simulink model "Controllers"  (R2022b)
settings: Solver=FixedStepAuto  StartTime=0.0  StopTime=60  FixedStep=.01  RelTol=1e-3
values from neighbouring files (symbols this model uses):
  g = [0, 0, 1]    [myMeasurementFcn.m]    (also in test_DELETE.m = [0,0,0,1])
undefined symbols (not defined in the file or in its folder): CdProp, Ct, larm, mass
libraries: slpidlib x6, sharedtransform x2
settings Model: Creator=aaron  LastModifiedBy=aaron
settings DataIOCC: SaveOutput=off  SaveTime=off
settings DebuggingCC: ModelReferenceExtraNoncontSigs=none

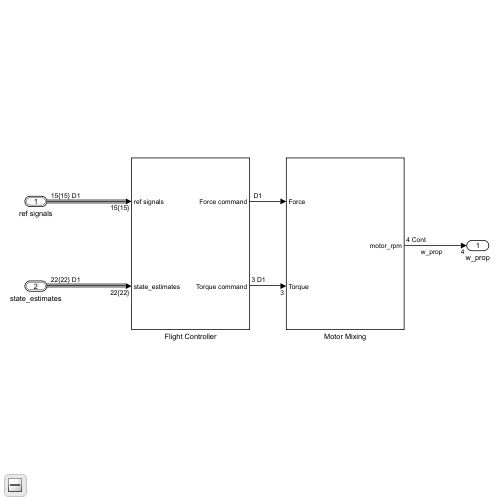
[thumbnail: Simulink's stored preview of the top-level diagram]
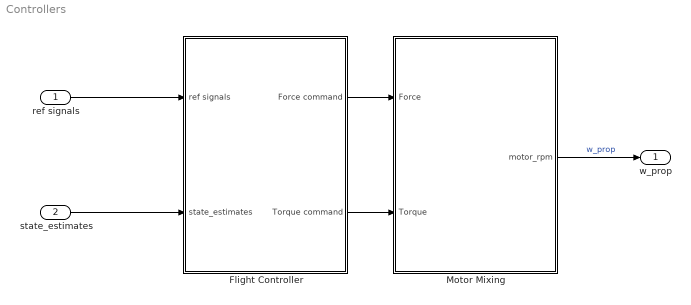
== system Controllers ==
  ref signals : Inport  OutDataTypeStr=Bus: reference_signals  SampleTime=[.01,0]  LockScale=on
  state_estimates : Inport  Port=2  OutDataTypeStr=Bus: state_estimates  SampleTime=[.01,0]  LockScale=on
  Flight Controller : Subsystem
  Motor Mixing : Subsystem
  w_prop : Outport  OutDataTypeStr=single  PortDimensions=4  SampleTime=0
  wires:
  state_estimates/1 -> Flight Controller/2(state_estimates)
  Motor Mixing/1(motor_rpm) -> w_prop/1  "w_prop"
  ref signals/1 -> Flight Controller/1(ref signals)
  Flight Controller/2(Torque command) -> Motor Mixing/2(Torque)
  Flight Controller/1(Force command) -> Motor Mixing/1(Force)

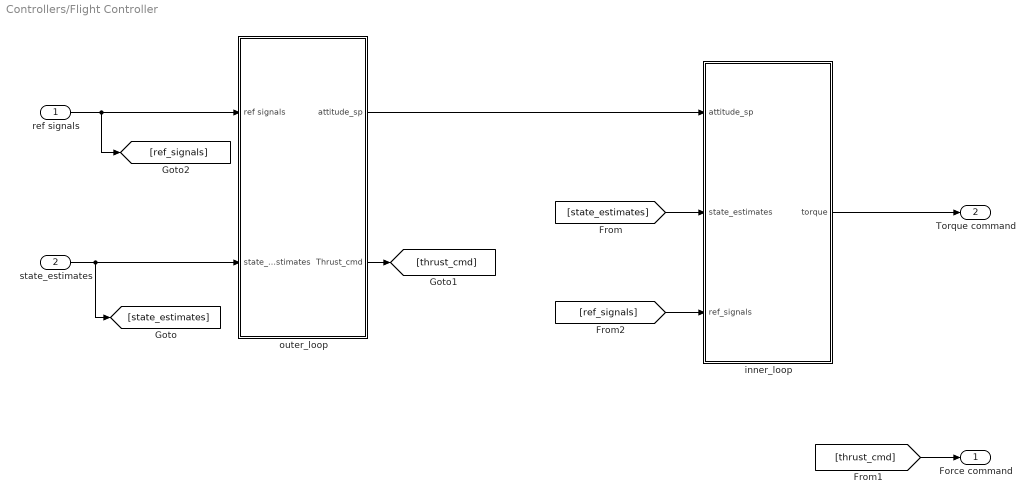
== system Controllers/Flight Controller ==
  ref signals : Inport  OutDataTypeStr=Bus: reference_signals  SampleTime=[.01,0]  LockScale=on
  state_estimates : Inport  Port=2  OutDataTypeStr=Bus: state_estimates  SampleTime=[.01,0]  LockScale=on
  inner_loop : Subsystem
  outer_loop : Subsystem
  Force command : Outport
  Torque command : Outport  Port=2
  wires:
  state_estimates/1 -> outer_loop/2(state_estimates), [state_estimates]
  ref signals/1 -> [ref_signals], outer_loop/1(ref signals)
  outer_loop/1(attitude_sp) -> inner_loop/1(attitude_sp)
  [state_estimates] -> inner_loop/2(state_estimates)
  inner_loop/1(torque) -> Torque command/1
  outer_loop/2(Thrust_cmd) -> [thrust_cmd]
  [thrust_cmd] -> Force command/1
  [ref_signals] -> inner_loop/3(ref_signals)

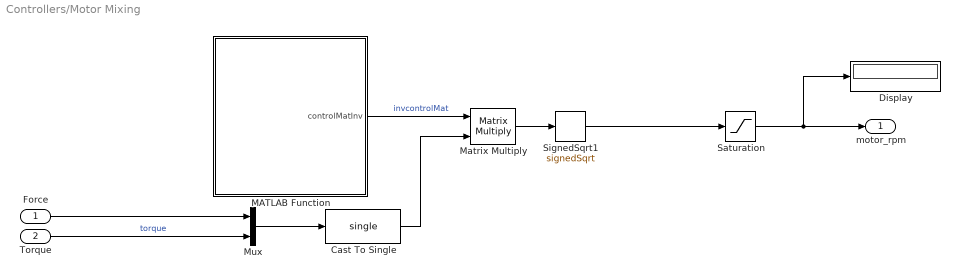
== system Controllers/Motor Mixing ==
  Force : Inport
  Torque : Inport  Port=2
  Cast To Single : DataTypeConversion  OutDataTypeStr=single  SaturateOnIntegerOverflow=off  RndMeth=Floor
  Display : Display
  MATLAB Function : MATLAB Function  TreatAsAtomicUnit=on
  Matrix Multiply : Product  Multiplication=Matrix(*)
  Mux : Mux  Inputs=2
  Saturation : Saturate  UpperLimit=2000  LowerLimit=0
  SignedSqrt1 : Sqrt  Operator=signedSqrt  IntermediateResultsDataTypeStr=single
  motor_rpm : Outport
  wires:
  Torque/1 -> Mux/2  "torque"
  Force/1 -> Mux/1
  Saturation/1 -> Display/1, motor_rpm/1
  SignedSqrt1/1 -> Saturation/1
  Matrix Multiply/1 -> SignedSqrt1/1
  MATLAB Function/1(controlMatInv) -> Matrix Multiply/1  "invcontrolMat"
  Cast To Single/1 -> Matrix Multiply/2
  Mux/1 -> Cast To Single/1

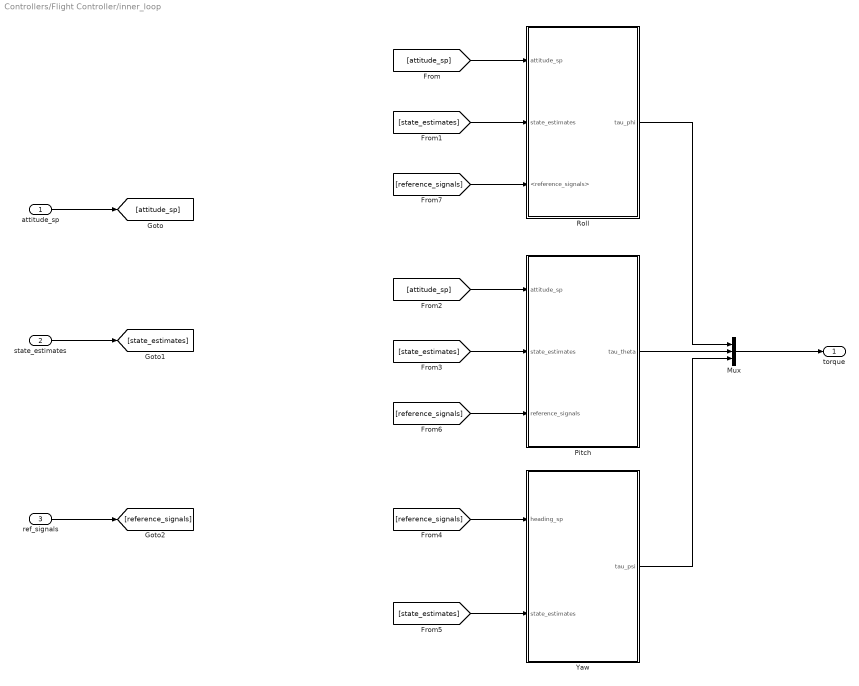
== system Controllers/Flight Controller/inner_loop ==
  attitude_sp : Inport
  state_estimates : Inport  Port=2  OutDataTypeStr=Bus: state_estimates  SampleTime=[.01,0]
  ref_signals : Inport  Port=3  OutDataTypeStr=Bus: reference_signals  SampleTime=[.01,0]
  Mux : Mux  Inputs=3
  Pitch : Subsystem
  Roll : Subsystem
  Yaw : Subsystem
  torque : Outport
  wires:
  [reference_signals] -> Roll/3(<reference_signals>)
  [reference_signals] -> Pitch/3(reference_signals)
  [reference_signals] -> Yaw/1(heading_sp)
  ref_signals/1 -> [reference_signals]
  attitude_sp/1 -> [attitude_sp]
  state_estimates/1 -> [state_estimates]
  [attitude_sp] -> Roll/1(attitude_sp)
  [state_estimates] -> Roll/2(state_estimates)
  [attitude_sp] -> Pitch/1(attitude_sp)
  [state_estimates] -> Pitch/2(state_estimates)
  [state_estimates] -> Yaw/2(state_estimates)
  Roll/1(tau_phi) -> Mux/1
  Mux/1 -> torque/1
  Pitch/1(tau_theta) -> Mux/2
  Yaw/1(tau_psi) -> Mux/3

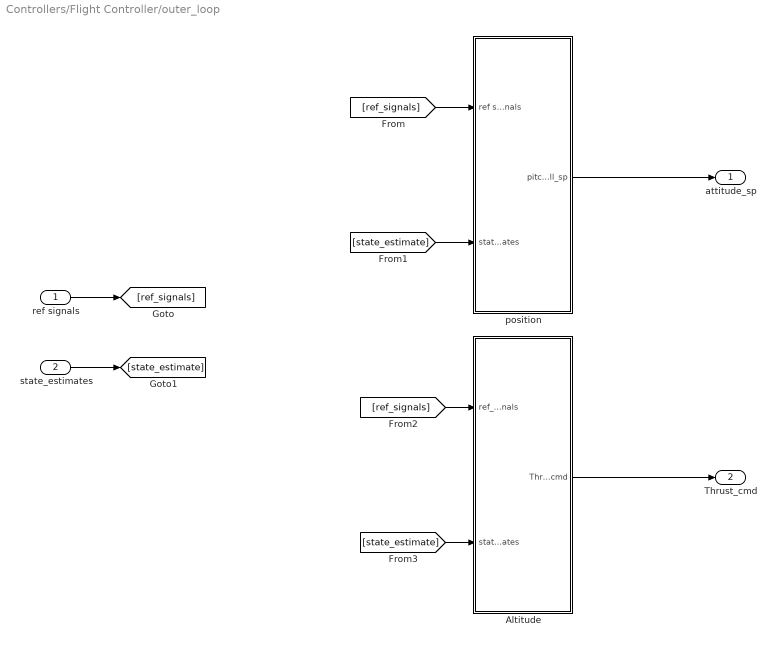
== system Controllers/Flight Controller/outer_loop ==
  ref signals : Inport  OutDataTypeStr=Bus: reference_signals  LockScale=on
  state_estimates : Inport  Port=2  OutDataTypeStr=Bus: state_estimates  LockScale=on
  Altitude : Subsystem
  position : Subsystem
  attitude_sp : Outport
  Thrust_cmd : Outport  Port=2
  wires:
  position/1(pitch_roll_sp) -> attitude_sp/1
  Altitude/1(Thrust_cmd) -> Thrust_cmd/1
  ref signals/1 -> [ref_signals]
  state_estimates/1 -> [state_estimate]
  [ref_signals] -> position/1(ref signals)
  [state_estimate] -> position/2(state_estimates)
  [ref_signals] -> Altitude/1(ref_signals)
  [state_estimate] -> Altitude/2(state_estimates)

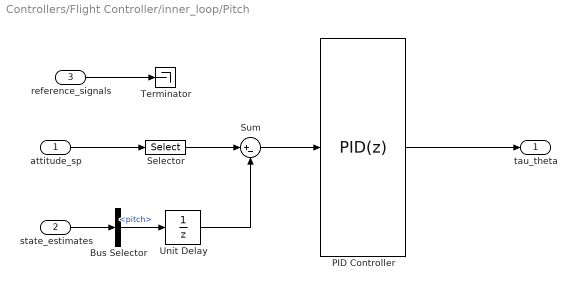
== system Controllers/Flight Controller/inner_loop/Pitch ==
  attitude_sp : Inport
  state_estimates : Inport  Port=2  OutDataTypeStr=Bus: state_estimates  SampleTime=[.01,0]
  reference_signals : Inport  Port=3  OutDataTypeStr=Bus: reference_signals  SampleTime=[.01,0]
  Bus Selector : BusSelector  OutputSignals=euler.pitch
  PID Controller : slpidlib/PID Controller  Controller=PID  Form=Parallel  TimeDomain=Discrete-time  UseExternalTs=off  SampleTime=-1  IntegratorMethod=Forward Euler  FilterMethod=Forward Euler  ControllerParametersSource=internal  P=0.000755  I=1.95e-05  UseKiTs=off  D=0.00509  N=1.0382  UseFilter=on  TunerSelectOption=Transfer Function Based (PID Tuner App)  InitialConditionSource=internal  InitialConditionForIntegrator=0  InitialConditionForFilter=0  DifferentiatorICPrevScaledInput=0  ExternalReset=none  TrackingMode=off  Kt=1  LimitOutput=off  SatLimitsSource=internal  UpperSaturationLimit=inf  LowerSaturationLimit=-inf  LinearizeAsGain=on  AntiWindupMode=clamping  Kb=1  LimitIntegrator=off  UpperIntegratorSaturationLimit=inf  LowerIntegratorSaturationLimit=-inf  POutMin=[]  POutMax=[]  IOutMin=[]  IOutMax=[]  DOutMin=[]  DOutMax=[]  NOutMin=[]  NOutMax=[]  SumOutMin=[]  SumOutMax=[]  SaturationOutMin=[]  SaturationOutMax=[]  PParamMin=[]  PParamMax=[]  IParamMin=[]  IParamMax=[]  DParamMin=[]  DParamMax=[]  NParamMin=[]  NParamMax=[]  KbParamMin=[]  KbParamMax=[]  KtParamMin=[]  KtParamMax=[]  KbOutMin=[]  KbOutMax=[]  KtOutMin=[]  KtOutMax=[]  IntegratorOutMin=[]  IntegratorOutMax=[]  FilterOutMin=[]  FilterOutMax=[]  SumI1OutMin=[]  SumI1OutMax=[]  SumI2OutMin=[]  SumI2OutMax=[]  SumI3OutMin=[]  SumI3OutMax=[]  SumI4OutMin=[]  SumI4OutMax=[]  SumDOutMin=[]  SumDOutMax=[]  DifferentiatorOutMin=[]  DifferentiatorOutMax=[]  FilterDiffOutCoefMin=[]  FilterDiffOutCoefMax=[]  ReciprocalOutMin=[]  ReciprocalOutMax=[]  SumDenOutMin=[]  SumDenOutMax=[]  SumNumOutMin=[]  SumNumOutMax=[]  DivideOutMin=[]  DivideOutMax=[]  UdiffTsProdOutMin=[]  UdiffTsProdOutMax=[]  NTsProdOutMin=[]  NTsProdOutMax=[]  UintegralTsProdOutMin=[]  UintegralTsProdOutMax=[]  UngainTsProdOutMin=[]  UngainTsProdOutMax=[]  ClampingZeroOutDataTypeStr=Inherit: Inherit via back propagation  ClampingZeroOutMin=[]  ClampingZeroOutMax=[]  FilterDenConstantOutDataTypeStr=Inherit: Inherit via back propagation  FilterDenConstantOutMin=[]  FilterDenConstantOutMax=[]  PCopyOutDataTypeStr=Inherit: Inherit via back propagation  PCopyOutMin=[]  PCopyOutMax=[]  NCopyOutDataTypeStr=Inherit: Inherit via back propagation  NCopyOutMin=[]  NCopyOutMax=[]  IntegratorContinuousStateAttributes=''  IntegratorStateMustResolveToSignalObject=off  IntegratorRTWStateStorageClass=Auto  FilterContinuousStateAttributes=''  FilterStateMustResolveToSignalObject=off  FilterRTWStateStorageClass=Auto  ParallelPVariant=InternalParameters  IdealPVariant=Disabled  IVariant=InternalParameters  DVariant=InternalParameters  IntegratorVariant=Discrete  SatVariant=Disabled  AWVariant=Passthrough  PCopyVariant=Disabled  TRVariant=Disabled  FdbkBlocksVariant=Forward  IdealPFdbkVariant=Disabled  SatFdbkVariant=Disabled  DerivativeFilterVariant=ForwardEulerFilter  NVariant=InternalParameters  NCopyVariant=Disabled  FilterICVariant=InternalICsFilter  IntegratorICVariant=InternalICs  ExternalResetVariant=Disabled  TRSumVariant=Passthrough  SumFdbkVariant=Disabled  SumVariant=Sum_PID  TsampFilterVariant=InternalTs  TsampNgainVariant=Passthrough  TsampIntegralVariant=Passthrough  ExternalSaturationOutDataTypeStr=Inherit: Same as second input
  Selector : Selector  InputPortWidth=2  IndexOptions=Index vector (dialog)  Indices=[2]  OutputSizes=1
  Sum : Sum  Inputs=|+-
  Terminator : Terminator
  Unit Delay : UnitDelay  InitialCondition=single(0)  SampleTime=-1  HasFrameUpgradeWarning=on
  tau_theta : Outport
  wires:
  attitude_sp/1 -> Selector/1
  Sum/1 -> PID Controller/1
  PID Controller/1 -> tau_theta/1
  Bus Selector/1 -> Unit Delay/1  "<pitch>"
  state_estimates/1 -> Bus Selector/1
  reference_signals/1 -> Terminator/1
  Selector/1 -> Sum/1
  Unit Delay/1 -> Sum/2

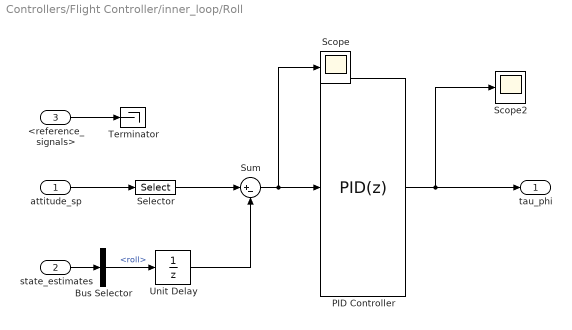
== system Controllers/Flight Controller/inner_loop/Roll ==
  attitude_sp : Inport
  state_estimates : Inport  Port=2  OutDataTypeStr=Bus: state_estimates
  <reference_signals> : Inport  Port=3  OutDataTypeStr=Bus: reference_signals
  Bus Selector : BusSelector  OutputSignals=euler.roll
  PID Controller : slpidlib/PID Controller  Controller=PID  Form=Parallel  TimeDomain=Discrete-time  UseExternalTs=off  SampleTime=-1  IntegratorMethod=Forward Euler  FilterMethod=Forward Euler  ControllerParametersSource=internal  P=0.00222776202264695  I=2.18485015437245e-05  UseKiTs=off  D=0.0134340999324703  N=1.24748629813611  UseFilter=on  TunerSelectOption=Transfer Function Based (PID Tuner App)  InitialConditionSource=internal  InitialConditionForIntegrator=0  InitialConditionForFilter=0  DifferentiatorICPrevScaledInput=0  ExternalReset=none  TrackingMode=off  Kt=1  LimitOutput=off  SatLimitsSource=internal  UpperSaturationLimit=inf  LowerSaturationLimit=-inf  LinearizeAsGain=on  AntiWindupMode=clamping  Kb=1  LimitIntegrator=off  UpperIntegratorSaturationLimit=inf  LowerIntegratorSaturationLimit=-inf  POutMin=[]  POutMax=[]  IOutMin=[]  IOutMax=[]  DOutMin=[]  DOutMax=[]  NOutMin=[]  NOutMax=[]  SumOutMin=[]  SumOutMax=[]  SaturationOutMin=[]  SaturationOutMax=[]  PParamMin=[]  PParamMax=[]  IParamMin=[]  IParamMax=[]  DParamMin=[]  DParamMax=[]  NParamMin=[]  NParamMax=[]  KbParamMin=[]  KbParamMax=[]  KtParamMin=[]  KtParamMax=[]  KbOutMin=[]  KbOutMax=[]  KtOutMin=[]  KtOutMax=[]  IntegratorOutMin=[]  IntegratorOutMax=[]  FilterOutMin=[]  FilterOutMax=[]  SumI1OutMin=[]  SumI1OutMax=[]  SumI2OutMin=[]  SumI2OutMax=[]  SumI3OutMin=[]  SumI3OutMax=[]  SumI4OutMin=[]  SumI4OutMax=[]  SumDOutMin=[]  SumDOutMax=[]  DifferentiatorOutMin=[]  DifferentiatorOutMax=[]  FilterDiffOutCoefMin=[]  FilterDiffOutCoefMax=[]  ReciprocalOutMin=[]  ReciprocalOutMax=[]  SumDenOutMin=[]  SumDenOutMax=[]  SumNumOutMin=[]  SumNumOutMax=[]  DivideOutMin=[]  DivideOutMax=[]  UdiffTsProdOutMin=[]  UdiffTsProdOutMax=[]  NTsProdOutMin=[]  NTsProdOutMax=[]  UintegralTsProdOutMin=[]  UintegralTsProdOutMax=[]  UngainTsProdOutMin=[]  UngainTsProdOutMax=[]  ClampingZeroOutDataTypeStr=Inherit: Inherit via back propagation  ClampingZeroOutMin=[]  ClampingZeroOutMax=[]  FilterDenConstantOutDataTypeStr=Inherit: Inherit via back propagation  FilterDenConstantOutMin=[]  FilterDenConstantOutMax=[]  PCopyOutDataTypeStr=Inherit: Inherit via back propagation  PCopyOutMin=[]  PCopyOutMax=[]  NCopyOutDataTypeStr=Inherit: Inherit via back propagation  NCopyOutMin=[]  NCopyOutMax=[]  IntegratorContinuousStateAttributes=''  IntegratorStateMustResolveToSignalObject=off  IntegratorRTWStateStorageClass=Auto  FilterContinuousStateAttributes=''  FilterStateMustResolveToSignalObject=off  FilterRTWStateStorageClass=Auto  ParallelPVariant=InternalParameters  IdealPVariant=Disabled  IVariant=InternalParameters  DVariant=InternalParameters  IntegratorVariant=Discrete  SatVariant=Disabled  AWVariant=Passthrough  PCopyVariant=Disabled  TRVariant=Disabled  FdbkBlocksVariant=Forward  IdealPFdbkVariant=Disabled  SatFdbkVariant=Disabled  DerivativeFilterVariant=ForwardEulerFilter  NVariant=InternalParameters  NCopyVariant=Disabled  FilterICVariant=InternalICsFilter  IntegratorICVariant=InternalICs  ExternalResetVariant=Disabled  TRSumVariant=Passthrough  SumFdbkVariant=Disabled  SumVariant=Sum_PID  TsampFilterVariant=InternalTs  TsampNgainVariant=Passthrough  TsampIntegralVariant=Passthrough  ExternalSaturationOutDataTypeStr=Inherit: Same as second input
  Scope : Scope
  Scope2 : Scope
  Selector : Selector  InputPortWidth=2  IndexOptions=Index vector (dialog)  Indices=[1]  OutputSizes=1
  Sum : Sum  Inputs=|+-
  Terminator : Terminator
  Unit Delay : UnitDelay  InitialCondition=single(0)  SampleTime=-1  HasFrameUpgradeWarning=on
  tau_phi : Outport
  wires:
  attitude_sp/1 -> Selector/1
  Sum/1 -> PID Controller/1, Scope/1
  PID Controller/1 -> Scope2/1, tau_phi/1
  state_estimates/1 -> Bus Selector/1
  Bus Selector/1 -> Unit Delay/1  "<roll>"
  <reference_signals>/1 -> Terminator/1
  Selector/1 -> Sum/1
  Unit Delay/1 -> Sum/2

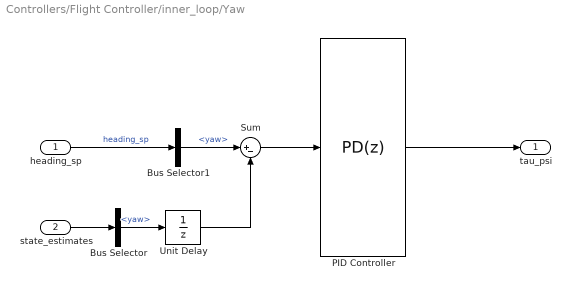
== system Controllers/Flight Controller/inner_loop/Yaw ==
  heading_sp : Inport  OutDataTypeStr=Bus: reference_signals
  state_estimates : Inport  Port=2  OutDataTypeStr=Bus: state_estimates
  Bus Selector : BusSelector  OutputSignals=euler.yaw
  Bus Selector1 : BusSelector  OutputSignals=euler.yaw
  PID Controller : slpidlib/PID Controller  Controller=PD  Form=Parallel  TimeDomain=Discrete-time  UseExternalTs=off  SampleTime=-1  IntegratorMethod=Forward Euler  FilterMethod=Forward Euler  ControllerParametersSource=internal  P=0.00308709400862221  I=0  UseKiTs=off  D=0.020762699011989  N=9.31948574377754  UseFilter=on  TunerSelectOption=Transfer Function Based (PID Tuner App)  InitialConditionSource=internal  InitialConditionForIntegrator=0  InitialConditionForFilter=0  DifferentiatorICPrevScaledInput=0  ExternalReset=none  TrackingMode=off  Kt=1  LimitOutput=off  SatLimitsSource=internal  UpperSaturationLimit=inf  LowerSaturationLimit=-inf  LinearizeAsGain=on  AntiWindupMode=clamping  Kb=1  LimitIntegrator=off  UpperIntegratorSaturationLimit=inf  LowerIntegratorSaturationLimit=-inf  POutMin=[]  POutMax=[]  IOutMin=[]  IOutMax=[]  DOutMin=[]  DOutMax=[]  NOutMin=[]  NOutMax=[]  SumOutMin=[]  SumOutMax=[]  SaturationOutMin=[]  SaturationOutMax=[]  PParamMin=[]  PParamMax=[]  IParamMin=[]  IParamMax=[]  DParamMin=[]  DParamMax=[]  NParamMin=[]  NParamMax=[]  KbParamMin=[]  KbParamMax=[]  KtParamMin=[]  KtParamMax=[]  KbOutMin=[]  KbOutMax=[]  KtOutMin=[]  KtOutMax=[]  IntegratorOutMin=[]  IntegratorOutMax=[]  FilterOutMin=[]  FilterOutMax=[]  SumI1OutMin=[]  SumI1OutMax=[]  SumI2OutMin=[]  SumI2OutMax=[]  SumI3OutMin=[]  SumI3OutMax=[]  SumI4OutMin=[]  SumI4OutMax=[]  SumDOutMin=[]  SumDOutMax=[]  DifferentiatorOutMin=[]  DifferentiatorOutMax=[]  FilterDiffOutCoefMin=[]  FilterDiffOutCoefMax=[]  ReciprocalOutMin=[]  ReciprocalOutMax=[]  SumDenOutMin=[]  SumDenOutMax=[]  SumNumOutMin=[]  SumNumOutMax=[]  DivideOutMin=[]  DivideOutMax=[]  UdiffTsProdOutMin=[]  UdiffTsProdOutMax=[]  NTsProdOutMin=[]  NTsProdOutMax=[]  UintegralTsProdOutMin=[]  UintegralTsProdOutMax=[]  UngainTsProdOutMin=[]  UngainTsProdOutMax=[]  ClampingZeroOutDataTypeStr=Inherit: Inherit via back propagation  ClampingZeroOutMin=[]  ClampingZeroOutMax=[]  FilterDenConstantOutDataTypeStr=Inherit: Inherit via back propagation  FilterDenConstantOutMin=[]  FilterDenConstantOutMax=[]  PCopyOutDataTypeStr=Inherit: Inherit via back propagation  PCopyOutMin=[]  PCopyOutMax=[]  NCopyOutDataTypeStr=Inherit: Inherit via back propagation  NCopyOutMin=[]  NCopyOutMax=[]  IntegratorContinuousStateAttributes=''  IntegratorStateMustResolveToSignalObject=off  IntegratorRTWStateStorageClass=Auto  FilterContinuousStateAttributes=''  FilterStateMustResolveToSignalObject=off  FilterRTWStateStorageClass=Auto  ParallelPVariant=InternalParameters  IdealPVariant=Disabled  IVariant=Disabled  DVariant=InternalParameters  IntegratorVariant=Disabled  SatVariant=Disabled  AWVariant=Disabled  PCopyVariant=Disabled  TRVariant=Disabled  FdbkBlocksVariant=Forward  IdealPFdbkVariant=Disabled  SatFdbkVariant=Disabled  DerivativeFilterVariant=ForwardEulerFilter  NVariant=InternalParameters  NCopyVariant=Disabled  FilterICVariant=InternalICsFilter  IntegratorICVariant=Disabled  ExternalResetVariant=Disabled  TRSumVariant=Passthrough  SumFdbkVariant=Disabled  SumVariant=Sum_PD  TsampFilterVariant=InternalTs  TsampNgainVariant=Passthrough  TsampIntegralVariant=Disabled_SignalSpec  ExternalSaturationOutDataTypeStr=Inherit: Same as second input
  Sum : Sum  Inputs=|+-
  Unit Delay : UnitDelay  InitialCondition=single(0)  SampleTime=-1  HasFrameUpgradeWarning=on
  tau_psi : Outport
  wires:
  heading_sp/1 -> Bus Selector1/1  "heading_sp"
  Bus Selector1/1 -> Sum/1  "<yaw>"
  PID Controller/1 -> tau_psi/1
  Bus Selector/1 -> Unit Delay/1  "<yaw>"
  state_estimates/1 -> Bus Selector/1
  Sum/1 -> PID Controller/1
  Unit Delay/1 -> Sum/2

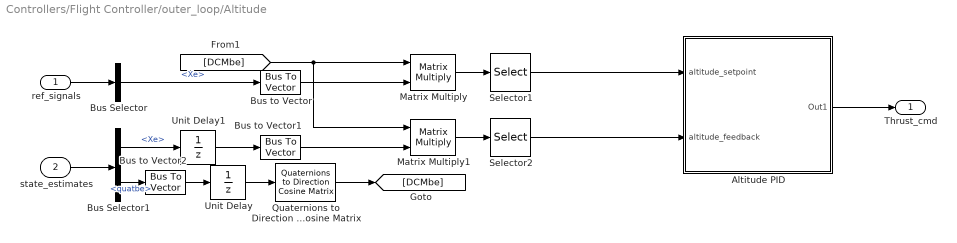
== system Controllers/Flight Controller/outer_loop/Altitude ==
  ref_signals : Inport  OutDataTypeStr=Bus: reference_signals  SampleTime=[.01,0]
  state_estimates : Inport  Port=2  OutDataTypeStr=Bus: state_estimates  SampleTime=[.01,0]
  Altitude PID : Subsystem
  Bus Selector : BusSelector  OutputSignals=Xe
  Bus Selector1 : BusSelector  OutputSignals=Xe,quatbe
  Bus to Vector : BusToVector
  Bus to Vector1 : BusToVector
  Bus to Vector2 : BusToVector
  Matrix Multiply : Product  Multiplication=Matrix(*)
  Matrix Multiply1 : Product  Multiplication=Matrix(*)
  Quaternions to Direction Cosine Matrix : sharedtransform/Quaternions to  Direction Cosine Matrix  aMode=aMode
      settings: LibrarySourceBlock=|
      | aerolibtransform2/Quaternions to
      | Direction Cosine Matrix
  Selector1 : Selector  InputPortWidth=3  IndexOptions=Index vector (dialog)  Indices=[3]  OutputSizes=1
  Selector2 : Selector  InputPortWidth=3  IndexOptions=Index vector (dialog)  Indices=[3]  OutputSizes=1
  Unit Delay : UnitDelay  InitialCondition=single([1,0,0,0])  SampleTime=-1  HasFrameUpgradeWarning=on
  Unit Delay1 : UnitDelay  InitialCondition=single([0,0,0])  SampleTime=-1  HasFrameUpgradeWarning=on
  Thrust_cmd : Outport
  wires:
  Quaternions to Direction Cosine Matrix/1 -> [DCMbe]
  Bus to Vector1/1 -> Matrix Multiply1/2
  Bus to Vector/1 -> Matrix Multiply/2
  Bus Selector1/1 -> Unit Delay1/1  "<Xe>"
  Bus Selector/1 -> Bus to Vector/1  "<Xe>"
  ref_signals/1 -> Bus Selector/1
  state_estimates/1 -> Bus Selector1/1
  Bus Selector1/2 -> Bus to Vector2/1  "<quatbe>"
  [DCMbe] -> Matrix Multiply1/1, Matrix Multiply/1
  Matrix Multiply1/1 -> Selector2/1
  Matrix Multiply/1 -> Selector1/1
  Selector1/1 -> Altitude PID/1(altitude_setpoint)
  Selector2/1 -> Altitude PID/2(altitude_feedback)
  Altitude PID/1(Out1) -> Thrust_cmd/1
  Bus to Vector2/1 -> Unit Delay/1
  Unit Delay/1 -> Quaternions to Direction Cosine Matrix/1
  Unit Delay1/1 -> Bus to Vector1/1

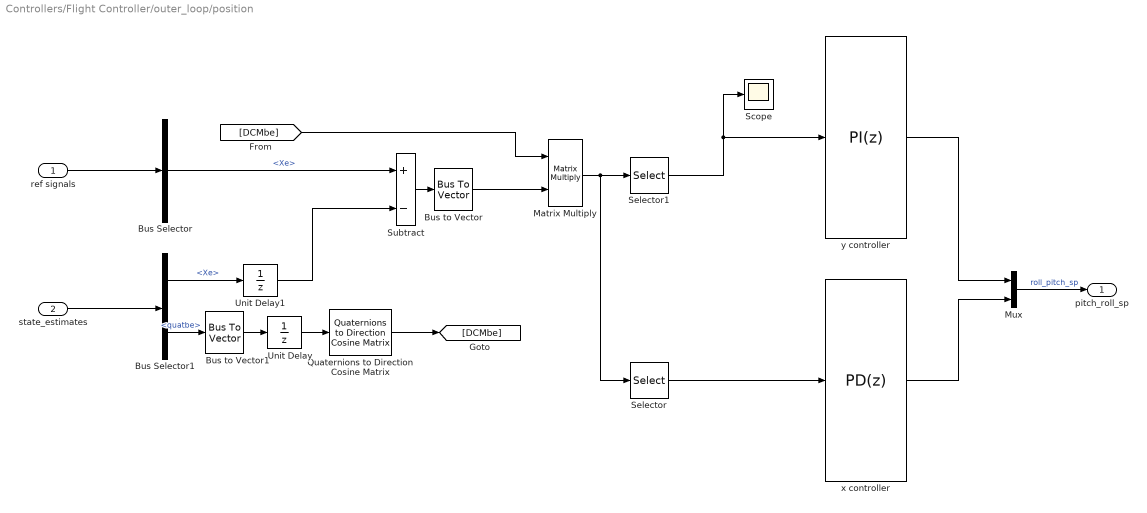
== system Controllers/Flight Controller/outer_loop/position ==
  ref signals : Inport  OutDataTypeStr=Bus: reference_signals  SampleTime=[.01,0]
  state_estimates : Inport  Port=2  OutDataTypeStr=Bus: state_estimates  SampleTime=[.01,0]
  Bus Selector : BusSelector  OutputSignals=Xe
  Bus Selector1 : BusSelector  OutputSignals=Xe,quatbe
  Bus to Vector : BusToVector
  Bus to Vector1 : BusToVector
  Matrix Multiply : Product  Multiplication=Matrix(*)
  Mux : Mux  Inputs=2
  Quaternions to Direction Cosine Matrix : sharedtransform/Quaternions to  Direction Cosine Matrix  aMode=aMode
      settings: LibrarySourceBlock=|
      | aerolibtransform2/Quaternions to
      | Direction Cosine Matrix
  Scope : Scope
  Selector : Selector  InputPortWidth=3  IndexOptions=Index vector (dialog)  Indices=[1]  OutputSizes=1
  Selector1 : Selector  InputPortWidth=3  IndexOptions=Index vector (dialog)  Indices=[2]  OutputSizes=1
  Subtract : Sum  Inputs=+-
  Unit Delay : UnitDelay  InitialCondition=single([1,0,0,0])  SampleTime=-1  HasFrameUpgradeWarning=on
  Unit Delay1 : UnitDelay  InitialCondition=single([0,0,0])  SampleTime=-1  HasFrameUpgradeWarning=on
  x controller : slpidlib/PID Controller  Controller=PD  Form=Parallel  TimeDomain=Discrete-time  UseExternalTs=off  SampleTime=-1  IntegratorMethod=Forward Euler  FilterMethod=Forward Euler  ControllerParametersSource=internal  P=-0.0205622316535753  I=.000001  UseKiTs=off  D=0  N=100  UseFilter=on  TunerSelectOption=Transfer Function Based (PID Tuner App)  InitialConditionSource=internal  InitialConditionForIntegrator=0  InitialConditionForFilter=0  DifferentiatorICPrevScaledInput=0  ExternalReset=none  TrackingMode=off  Kt=1  LimitOutput=off  SatLimitsSource=internal  UpperSaturationLimit=inf  LowerSaturationLimit=-inf  LinearizeAsGain=on  AntiWindupMode=clamping  Kb=1  LimitIntegrator=off  UpperIntegratorSaturationLimit=inf  LowerIntegratorSaturationLimit=-inf  POutMin=[]  POutMax=[]  IOutMin=[]  IOutMax=[]  DOutMin=[]  DOutMax=[]  NOutMin=[]  NOutMax=[]  SumOutMin=[]  SumOutMax=[]  SaturationOutMin=[]  SaturationOutMax=[]  PParamMin=[]  PParamMax=[]  IParamMin=[]  IParamMax=[]  DParamMin=[]  DParamMax=[]  NParamMin=[]  NParamMax=[]  KbParamMin=[]  KbParamMax=[]  KtParamMin=[]  KtParamMax=[]  KbOutMin=[]  KbOutMax=[]  KtOutMin=[]  KtOutMax=[]  IntegratorOutMin=[]  IntegratorOutMax=[]  FilterOutMin=[]  FilterOutMax=[]  SumI1OutMin=[]  SumI1OutMax=[]  SumI2OutMin=[]  SumI2OutMax=[]  SumI3OutMin=[]  SumI3OutMax=[]  SumI4OutMin=[]  SumI4OutMax=[]  SumDOutMin=[]  SumDOutMax=[]  DifferentiatorOutMin=[]  DifferentiatorOutMax=[]  FilterDiffOutCoefMin=[]  FilterDiffOutCoefMax=[]  ReciprocalOutMin=[]  ReciprocalOutMax=[]  SumDenOutMin=[]  SumDenOutMax=[]  SumNumOutMin=[]  SumNumOutMax=[]  DivideOutMin=[]  DivideOutMax=[]  UdiffTsProdOutMin=[]  UdiffTsProdOutMax=[]  NTsProdOutMin=[]  NTsProdOutMax=[]  UintegralTsProdOutMin=[]  UintegralTsProdOutMax=[]  UngainTsProdOutMin=[]  UngainTsProdOutMax=[]  ClampingZeroOutDataTypeStr=Inherit: Inherit via back propagation  ClampingZeroOutMin=[]  ClampingZeroOutMax=[]  FilterDenConstantOutDataTypeStr=Inherit: Inherit via back propagation  FilterDenConstantOutMin=[]  FilterDenConstantOutMax=[]  PCopyOutDataTypeStr=Inherit: Inherit via back propagation  PCopyOutMin=[]  PCopyOutMax=[]  NCopyOutDataTypeStr=Inherit: Inherit via back propagation  NCopyOutMin=[]  NCopyOutMax=[]  IntegratorContinuousStateAttributes=''  IntegratorStateMustResolveToSignalObject=off  IntegratorRTWStateStorageClass=Auto  FilterContinuousStateAttributes=''  FilterStateMustResolveToSignalObject=off  FilterRTWStateStorageClass=Auto  ParallelPVariant=InternalParameters  IdealPVariant=Disabled  IVariant=Disabled  DVariant=InternalParameters  IntegratorVariant=Disabled  SatVariant=Disabled  AWVariant=Disabled  PCopyVariant=Disabled  TRVariant=Disabled  FdbkBlocksVariant=Forward  IdealPFdbkVariant=Disabled  SatFdbkVariant=Disabled  DerivativeFilterVariant=ForwardEulerFilter  NVariant=InternalParameters  NCopyVariant=Disabled  FilterICVariant=InternalICsFilter  IntegratorICVariant=Disabled  ExternalResetVariant=Disabled  TRSumVariant=Passthrough  SumFdbkVariant=Disabled  SumVariant=Sum_PD  TsampFilterVariant=InternalTs  TsampNgainVariant=Passthrough  TsampIntegralVariant=Disabled_SignalSpec  ExternalSaturationOutDataTypeStr=Inherit: Same as second input
  y controller : slpidlib/PID Controller  Controller=PI  Form=Parallel  TimeDomain=Discrete-time  UseExternalTs=off  SampleTime=-1  IntegratorMethod=Forward Euler  FilterMethod=Forward Euler  ControllerParametersSource=internal  P=0.0214287173644059  I=8.55230649524744e-05  UseKiTs=off  D=0  N=100  UseFilter=on  TunerSelectOption=Transfer Function Based (PID Tuner App)  InitialConditionSource=internal  InitialConditionForIntegrator=0  InitialConditionForFilter=0  DifferentiatorICPrevScaledInput=0  ExternalReset=none  TrackingMode=off  Kt=1  LimitOutput=off  SatLimitsSource=internal  UpperSaturationLimit=inf  LowerSaturationLimit=-inf  LinearizeAsGain=on  AntiWindupMode=clamping  Kb=1  LimitIntegrator=off  UpperIntegratorSaturationLimit=inf  LowerIntegratorSaturationLimit=-inf  POutMin=[]  POutMax=[]  IOutMin=[]  IOutMax=[]  DOutMin=[]  DOutMax=[]  NOutMin=[]  NOutMax=[]  SumOutMin=[]  SumOutMax=[]  SaturationOutMin=[]  SaturationOutMax=[]  PParamMin=[]  PParamMax=[]  IParamMin=[]  IParamMax=[]  DParamMin=[]  DParamMax=[]  NParamMin=[]  NParamMax=[]  KbParamMin=[]  KbParamMax=[]  KtParamMin=[]  KtParamMax=[]  KbOutMin=[]  KbOutMax=[]  KtOutMin=[]  KtOutMax=[]  IntegratorOutMin=[]  IntegratorOutMax=[]  FilterOutMin=[]  FilterOutMax=[]  SumI1OutMin=[]  SumI1OutMax=[]  SumI2OutMin=[]  SumI2OutMax=[]  SumI3OutMin=[]  SumI3OutMax=[]  SumI4OutMin=[]  SumI4OutMax=[]  SumDOutMin=[]  SumDOutMax=[]  DifferentiatorOutMin=[]  DifferentiatorOutMax=[]  FilterDiffOutCoefMin=[]  FilterDiffOutCoefMax=[]  ReciprocalOutMin=[]  ReciprocalOutMax=[]  SumDenOutMin=[]  SumDenOutMax=[]  SumNumOutMin=[]  SumNumOutMax=[]  DivideOutMin=[]  DivideOutMax=[]  UdiffTsProdOutMin=[]  UdiffTsProdOutMax=[]  NTsProdOutMin=[]  NTsProdOutMax=[]  UintegralTsProdOutMin=[]  UintegralTsProdOutMax=[]  UngainTsProdOutMin=[]  UngainTsProdOutMax=[]  ClampingZeroOutDataTypeStr=Inherit: Inherit via back propagation  ClampingZeroOutMin=[]  ClampingZeroOutMax=[]  FilterDenConstantOutDataTypeStr=Inherit: Inherit via back propagation  FilterDenConstantOutMin=[]  FilterDenConstantOutMax=[]  PCopyOutDataTypeStr=Inherit: Inherit via back propagation  PCopyOutMin=[]  PCopyOutMax=[]  NCopyOutDataTypeStr=Inherit: Inherit via back propagation  NCopyOutMin=[]  NCopyOutMax=[]  IntegratorContinuousStateAttributes=''  IntegratorStateMustResolveToSignalObject=off  IntegratorRTWStateStorageClass=Auto  FilterContinuousStateAttributes=''  FilterStateMustResolveToSignalObject=off  FilterRTWStateStorageClass=Auto  ParallelPVariant=InternalParameters  IdealPVariant=Disabled  IVariant=InternalParameters  DVariant=Disabled  IntegratorVariant=Discrete  SatVariant=Disabled  AWVariant=Passthrough  PCopyVariant=Disabled  TRVariant=Disabled  FdbkBlocksVariant=Forward  IdealPFdbkVariant=Disabled  SatFdbkVariant=Disabled  DerivativeFilterVariant=Disabled  NVariant=Disabled  NCopyVariant=Disabled_SignalSpec  FilterICVariant=Disabled  IntegratorICVariant=InternalICs  ExternalResetVariant=Disabled  TRSumVariant=Passthrough  SumFdbkVariant=Disabled  SumVariant=Sum_PI  TsampFilterVariant=InternalTs  TsampNgainVariant=Passthrough  TsampIntegralVariant=Passthrough  ExternalSaturationOutDataTypeStr=Inherit: Same as second input
  pitch_roll_sp : Outport
  wires:
  Quaternions to Direction Cosine Matrix/1 -> [DCMbe]
  Bus to Vector/1 -> Matrix Multiply/2
  Subtract/1 -> Bus to Vector/1
  ref signals/1 -> Bus Selector/1
  state_estimates/1 -> Bus Selector1/1
  Bus Selector/1 -> Subtract/1  "<Xe>"
  Bus Selector1/1 -> Unit Delay1/1  "<Xe>"
  [DCMbe] -> Matrix Multiply/1
  Bus Selector1/2 -> Bus to Vector1/1  "<quatbe>"
  Matrix Multiply/1 -> Selector1/1, Selector/1
  Selector/1 -> x controller/1
  Selector1/1 -> y controller/1, Scope/1
  Mux/1 -> pitch_roll_sp/1  "roll_pitch_sp"
  x controller/1 -> Mux/2
  y controller/1 -> Mux/1
  Unit Delay/1 -> Quaternions to Direction Cosine Matrix/1
  Bus to Vector1/1 -> Unit Delay/1
  Unit Delay1/1 -> Subtract/2

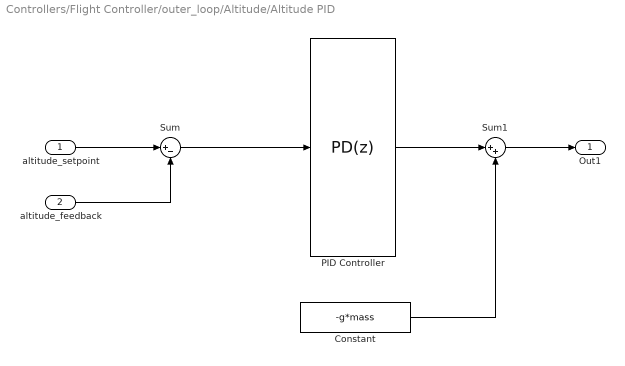
== system Controllers/Flight Controller/outer_loop/Altitude/Altitude PID ==
  altitude_setpoint : Inport
  altitude_feedback : Inport  Port=2
  Constant : Constant  Value=-g*mass
  PID Controller : slpidlib/PID Controller  Controller=PD  Form=Parallel  TimeDomain=Discrete-time  UseExternalTs=off  SampleTime=-1  IntegratorMethod=Forward Euler  FilterMethod=Forward Euler  ControllerParametersSource=internal  P=0.391711979722748  I=0  UseKiTs=off  D=0.101719151159153  N=0.643160901514191  UseFilter=on  TunerSelectOption=Transfer Function Based (PID Tuner App)  InitialConditionSource=internal  InitialConditionForIntegrator=0  InitialConditionForFilter=0  DifferentiatorICPrevScaledInput=0  ExternalReset=none  TrackingMode=off  Kt=1  LimitOutput=off  SatLimitsSource=internal  UpperSaturationLimit=inf  LowerSaturationLimit=-inf  LinearizeAsGain=on  AntiWindupMode=clamping  Kb=1  LimitIntegrator=off  UpperIntegratorSaturationLimit=inf  LowerIntegratorSaturationLimit=-inf  POutMin=[]  POutMax=[]  IOutMin=[]  IOutMax=[]  DOutMin=[]  DOutMax=[]  NOutMin=[]  NOutMax=[]  SumOutMin=[]  SumOutMax=[]  SaturationOutMin=[]  SaturationOutMax=[]  PParamMin=[]  PParamMax=[]  IParamMin=[]  IParamMax=[]  DParamMin=[]  DParamMax=[]  NParamMin=[]  NParamMax=[]  KbParamMin=[]  KbParamMax=[]  KtParamMin=[]  KtParamMax=[]  KbOutMin=[]  KbOutMax=[]  KtOutMin=[]  KtOutMax=[]  IntegratorOutMin=[]  IntegratorOutMax=[]  FilterOutMin=[]  FilterOutMax=[]  SumI1OutMin=[]  SumI1OutMax=[]  SumI2OutMin=[]  SumI2OutMax=[]  SumI3OutMin=[]  SumI3OutMax=[]  SumI4OutMin=[]  SumI4OutMax=[]  SumDOutMin=[]  SumDOutMax=[]  DifferentiatorOutMin=[]  DifferentiatorOutMax=[]  FilterDiffOutCoefMin=[]  FilterDiffOutCoefMax=[]  ReciprocalOutMin=[]  ReciprocalOutMax=[]  SumDenOutMin=[]  SumDenOutMax=[]  SumNumOutMin=[]  SumNumOutMax=[]  DivideOutMin=[]  DivideOutMax=[]  UdiffTsProdOutMin=[]  UdiffTsProdOutMax=[]  NTsProdOutMin=[]  NTsProdOutMax=[]  UintegralTsProdOutMin=[]  UintegralTsProdOutMax=[]  UngainTsProdOutMin=[]  UngainTsProdOutMax=[]  ClampingZeroOutDataTypeStr=Inherit: Inherit via back propagation  ClampingZeroOutMin=[]  ClampingZeroOutMax=[]  FilterDenConstantOutDataTypeStr=Inherit: Inherit via back propagation  FilterDenConstantOutMin=[]  FilterDenConstantOutMax=[]  PCopyOutDataTypeStr=Inherit: Inherit via back propagation  PCopyOutMin=[]  PCopyOutMax=[]  NCopyOutDataTypeStr=Inherit: Inherit via back propagation  NCopyOutMin=[]  NCopyOutMax=[]  IntegratorContinuousStateAttributes=''  IntegratorStateMustResolveToSignalObject=off  IntegratorRTWStateStorageClass=Auto  FilterContinuousStateAttributes=''  FilterStateMustResolveToSignalObject=off  FilterRTWStateStorageClass=Auto  ParallelPVariant=InternalParameters  IdealPVariant=Disabled  IVariant=Disabled  DVariant=InternalParameters  IntegratorVariant=Disabled  SatVariant=Disabled  AWVariant=Disabled  PCopyVariant=Disabled  TRVariant=Disabled  FdbkBlocksVariant=Forward  IdealPFdbkVariant=Disabled  SatFdbkVariant=Disabled  DerivativeFilterVariant=ForwardEulerFilter  NVariant=InternalParameters  NCopyVariant=Disabled  FilterICVariant=InternalICsFilter  IntegratorICVariant=Disabled  ExternalResetVariant=Disabled  TRSumVariant=Passthrough  SumFdbkVariant=Disabled  SumVariant=Sum_PD  TsampFilterVariant=InternalTs  TsampNgainVariant=Passthrough  TsampIntegralVariant=Disabled_SignalSpec  ExternalSaturationOutDataTypeStr=Inherit: Same as second input
  Sum : Sum  Inputs=|+-
  Sum1 : Sum  Inputs=|++
  Out1 : Outport
  wires:
  Sum/1 -> PID Controller/1
  PID Controller/1 -> Sum1/1
  Constant/1 -> Sum1/2
  altitude_feedback/1 -> Sum/2
  Sum1/1 -> Out1/1
  altitude_setpoint/1 -> Sum/1

== matlab function Controllers/Motor Mixing/MATLAB Function ==
  data: controlMatInv output; Ct parameter; larm parameter; CdProp parameter
function controlMatInv = calc_motor_speed(Ct,...
larm, CdProp)
% u1 = force;
% u2 = torques(1);
% u3 = torques(2);
% u4 = torques(3);


K = Ct;
L = larm;
C = CdProp;

% invControlMat = -[(C*u2 + C*u3 + C*L*u1 + K*L*u4)/(4*C*K*L);
%  (C*u2 - C*u3 - C*L*u1 + K*L*u4)/(4*C*K*L);
%  (C*u2 + C*u3 - C*L*u1 - K*L*u4)/(4*C*K*L);
% -(C*u2 - C*u3 + C*L*u1 - K*L*u4)/(4*C*K*L)];

invControlMat = [-1/(4*K), -1/(4*K*L), -1/(4*K*L), -1/(4*C);
                -1/(4*K),  1/(4*K*L), -1/(4*K*L),  1/(4*C);
                -1/(4*K),  1/(4*K*L),  1/(4*K*L), -1/(4*C);
                -1/(4*K), -1/(4*K*L),  1/(4*K*L),  1/(4*C)];
controlMatInv = invControlMat;
